simulink model "kiem_chung_dong_hoc"  (R2021a)
settings: Solver=FixedStepAuto  StartTime=0.0  StopTime=5  FixedStep=0.01  RelTol=1e-3
values from neighbouring files (symbols this model uses):
  X = Toado(:,1)    [QuydaoK.m]
  Y = Toado(:,2)    [QuydaoK.m]
  Z = Toado(:,3)    [QuydaoK.m]
undefined symbols (not defined in the file or in its folder): smiData
libraries: sm_lib x36, nesl_utility x13, simulink_extras x12
(part 1 of 4)
settings Model: Creator=ASUS  LastModifiedBy=NGAI-LAPTOP
settings SolverCC: AlgebraicLoopSolver=TrustRegion
settings DataIOCC: ReturnWorkspaceOutputs=off
settings SFSimCC: CustomCodeUndefinedFunction=UseInterfaceOnly
settings RTWCC: DLArmComputeVersion=20.02.1

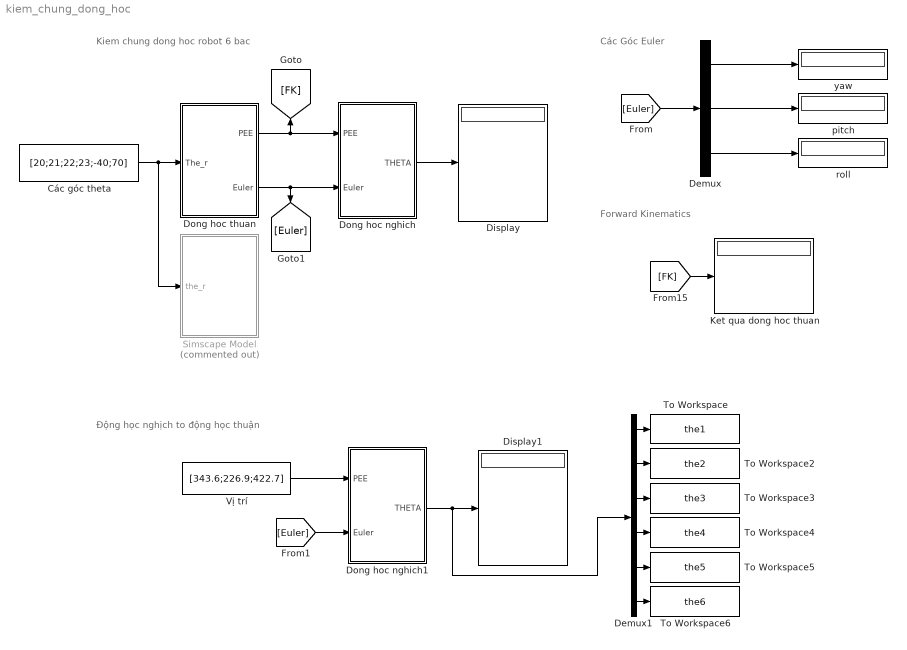
== system kiem_chung_dong_hoc ==
  note: Động học nghịch to động học thuận
  note: Kiem chung dong hoc robot 6 bac
  note: Forward Kinematics
  note: Các Góc Euler
  Các góc theta : Constant  Value=[20;21;22;23;-40;70]
  Demux : Demux  Outputs=3
  Demux1 : Demux  Outputs=6
  Display : Display
  Display1 : Display
  Dong hoc nghich : Subsystem
  Dong hoc nghich1 : Subsystem
  Dong hoc thuan : Subsystem
  Ket qua dong hoc thuan : Display
  Simscape Model : Subsystem  Commented=on
      mask Display: image('D:\Pictures\z4457172894230_43217be1eddd065875be42e85f2d9fb9.jpg');
  To Workspace : ToWorkspace  VariableName=the1  SaveFormat=Timeseries  SampleTime=-1
  To Workspace2 : ToWorkspace  VariableName=the2  SaveFormat=Timeseries  SampleTime=-1
  To Workspace3 : ToWorkspace  VariableName=the3  SaveFormat=Timeseries  SampleTime=-1
  To Workspace4 : ToWorkspace  VariableName=the4  SaveFormat=Timeseries  SampleTime=-1
  To Workspace5 : ToWorkspace  VariableName=the5  SaveFormat=Timeseries  SampleTime=-1
  To Workspace6 : ToWorkspace  VariableName=the6  SaveFormat=Timeseries  SampleTime=-1
  Vị trí : Constant  Value=[343.6;226.9;422.7]
  pitch : Display
  roll : Display
  yaw : Display
  wires:
  Demux/1 -> yaw/1
  Demux/2 -> pitch/1
  Demux/3 -> roll/1
  [FK] -> Ket qua dong hoc thuan/1
  Dong hoc thuan/1(PEE) -> Dong hoc nghich/1(PEE), [FK]
  Các góc theta/1 -> Simscape Model/1("the_r "), Dong hoc thuan/1(The_r)
  Dong hoc thuan/2(Euler) -> Dong hoc nghich/2(Euler), [Euler]
  [Euler] -> Demux/1
  Dong hoc nghich/1(THETA) -> Display/1
  [Euler] -> Dong hoc nghich1/2(Euler)
  Vị trí/1 -> Dong hoc nghich1/1(PEE)
  Demux1/5 -> To Workspace5/1
  Demux1/3 -> To Workspace3/1
  Demux1/4 -> To Workspace4/1
  Dong hoc nghich1/1(THETA) -> Demux1/1, Display1/1
  Demux1/2 -> To Workspace2/1
  Demux1/1 -> To Workspace/1
  Demux1/6 -> To Workspace6/1

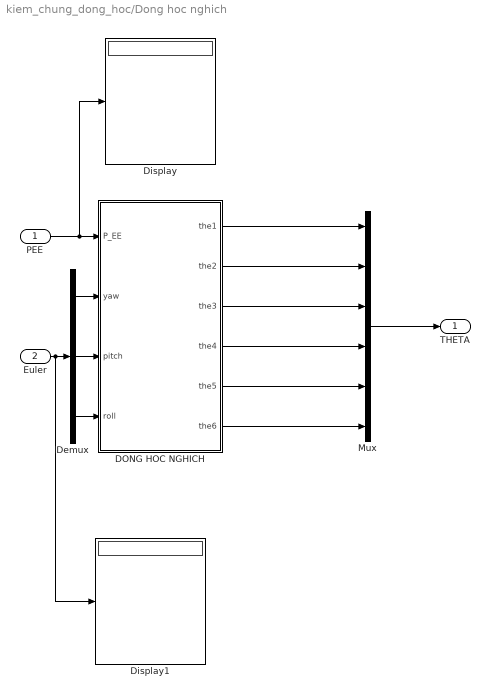
== system kiem_chung_dong_hoc/Dong hoc nghich ==
  PEE : Inport
  Euler : Inport  Port=2
  DONG HOC NGHICH : MATLAB Function  TreatAsAtomicUnit=on
  Demux : Demux  Outputs=3
  Display : Display
  Display1 : Display
  Mux : Mux  Inputs=6
  THETA : Outport
  wires:
  Demux/3 -> DONG HOC NGHICH/4(roll)
  Demux/1 -> DONG HOC NGHICH/2(yaw)
  Demux/2 -> DONG HOC NGHICH/3(pitch)
  DONG HOC NGHICH/3(the3) -> Mux/3
  DONG HOC NGHICH/4(the4) -> Mux/4
  DONG HOC NGHICH/2(the2) -> Mux/2
  DONG HOC NGHICH/6(the6) -> Mux/6
  DONG HOC NGHICH/5(the5) -> Mux/5
  PEE/1 -> Display/1, DONG HOC NGHICH/1(P_EE)
  Euler/1 -> Display1/1, Demux/1
  DONG HOC NGHICH/1(the1) -> Mux/1
  Mux/1 -> THETA/1

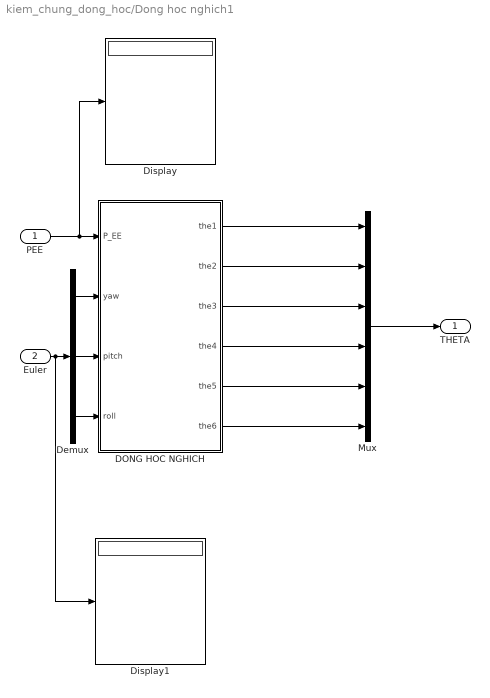
== system kiem_chung_dong_hoc/Dong hoc nghich1 ==
  PEE : Inport
  Euler : Inport  Port=2
  DONG HOC NGHICH : MATLAB Function  TreatAsAtomicUnit=on
  Demux : Demux  Outputs=3
  Display : Display
  Display1 : Display
  Mux : Mux  Inputs=6
  THETA : Outport
  wires:
  Demux/3 -> DONG HOC NGHICH/4(roll)
  Demux/1 -> DONG HOC NGHICH/2(yaw)
  Demux/2 -> DONG HOC NGHICH/3(pitch)
  DONG HOC NGHICH/3(the3) -> Mux/3
  DONG HOC NGHICH/4(the4) -> Mux/4
  DONG HOC NGHICH/2(the2) -> Mux/2
  DONG HOC NGHICH/6(the6) -> Mux/6
  DONG HOC NGHICH/5(the5) -> Mux/5
  PEE/1 -> Display/1, DONG HOC NGHICH/1(P_EE)
  Euler/1 -> Display1/1, Demux/1
  DONG HOC NGHICH/1(the1) -> Mux/1
  Mux/1 -> THETA/1

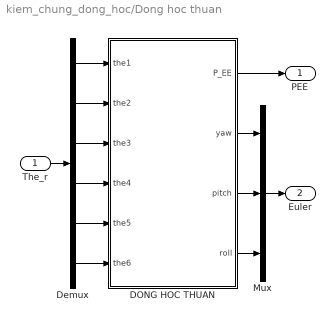
== system kiem_chung_dong_hoc/Dong hoc thuan ==
  The_r : Inport
  DONG HOC THUAN : MATLAB Function  TreatAsAtomicUnit=on
  Demux : Demux  Outputs=6
  Mux : Mux  Inputs=3
  PEE : Outport  VectorParamsAs1DForOutWhenUnconnected=off
  Euler : Outport  Port=2  VectorParamsAs1DForOutWhenUnconnected=off
  wires:
  Demux/5 -> DONG HOC THUAN/5(the5)
  Demux/1 -> DONG HOC THUAN/1(the1)
  Demux/4 -> DONG HOC THUAN/4(the4)
  DONG HOC THUAN/4(roll) -> Mux/3
  Demux/2 -> DONG HOC THUAN/2(the2)
  Demux/3 -> DONG HOC THUAN/3(the3)
  Demux/6 -> DONG HOC THUAN/6(the6)
  The_r/1 -> Demux/1
  DONG HOC THUAN/2(yaw) -> Mux/1
  DONG HOC THUAN/3(pitch) -> Mux/2
  Mux/1 -> Euler/1
  DONG HOC THUAN/1(P_EE) -> PEE/1
